simulink model "EngPrt"  (R2018a)
settings: configuration reference "cs_ert" (kept outside this file)
settings Model: DataDictionary=EngPrt.sldd  Creator=zhoutinglin  LastModifiedBy=zhoutinglin

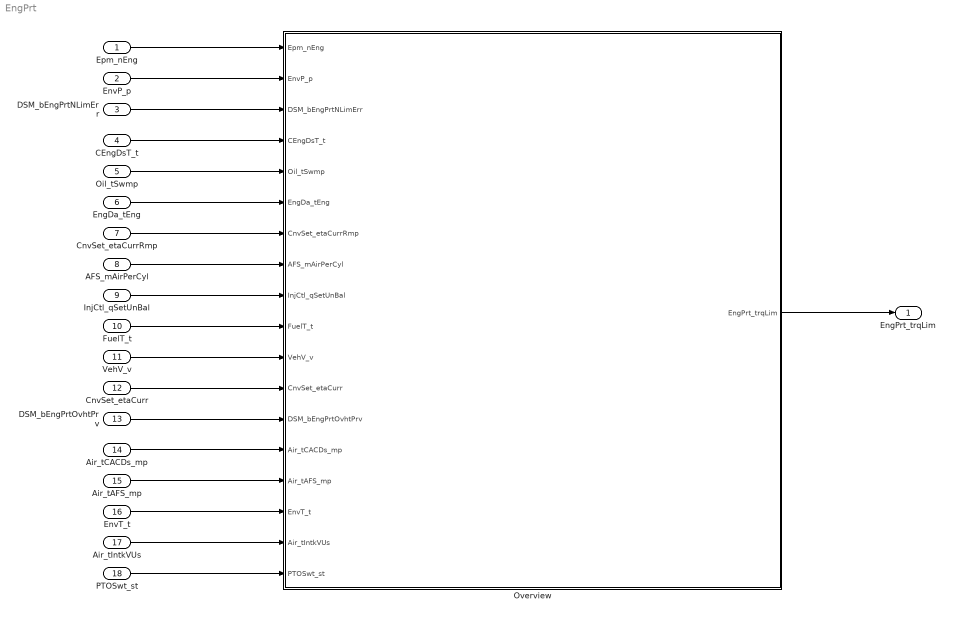
== system EngPrt ==
  Epm_nEng : Inport
  EnvP_p : Inport  Port=2
  DSM_bEngPrtNLimErr : Inport  Port=3
  CEngDsT_t : Inport  Port=4
  Oil_tSwmp : Inport  Port=5
  EngDa_tEng : Inport  Port=6
  CnvSet_etaCurrRmp : Inport  Port=7
  AFS_mAirPerCyl : Inport  Port=8
  InjCtl_qSetUnBal : Inport  Port=9
  FuelT_t : Inport  Port=10
  VehV_v : Inport  Port=11
  CnvSet_etaCurr : Inport  Port=12
  DSM_bEngPrtOvhtPrv : Inport  Port=13
  Air_tCACDs_mp : Inport  Port=14
  Air_tAFS_mp : Inport  Port=15
  EnvT_t : Inport  Port=16
  Air_tIntkVUs : Inport  Port=17
  PTOSwt_st : Inport  Port=18
  Overview : Subsystem
  EngPrt_trqLim : Outport
  wires:
  Epm_nEng/1 -> Overview/1(Epm_nEng)
  EnvP_p/1 -> Overview/2(EnvP_p)
  DSM_bEngPrtNLimErr/1 -> Overview/3(DSM_bEngPrtNLimErr)
  CEngDsT_t/1 -> Overview/4(CEngDsT_t)
  Oil_tSwmp/1 -> Overview/5(Oil_tSwmp)
  EngDa_tEng/1 -> Overview/6(EngDa_tEng)
  CnvSet_etaCurrRmp/1 -> Overview/7(CnvSet_etaCurrRmp)
  AFS_mAirPerCyl/1 -> Overview/8(AFS_mAirPerCyl)
  InjCtl_qSetUnBal/1 -> Overview/9(InjCtl_qSetUnBal)
  FuelT_t/1 -> Overview/10(FuelT_t)
  VehV_v/1 -> Overview/11(VehV_v)
  CnvSet_etaCurr/1 -> Overview/12(CnvSet_etaCurr)
  DSM_bEngPrtOvhtPrv/1 -> Overview/13(DSM_bEngPrtOvhtPrv)
  Air_tCACDs_mp/1 -> Overview/14(Air_tCACDs_mp)
  Air_tAFS_mp/1 -> Overview/15(Air_tAFS_mp)
  EnvT_t/1 -> Overview/16(EnvT_t)
  Air_tIntkVUs/1 -> Overview/17(Air_tIntkVUs)
  PTOSwt_st/1 -> Overview/18(PTOSwt_st)
  Overview/1(EngPrt_trqLim) -> EngPrt_trqLim/1

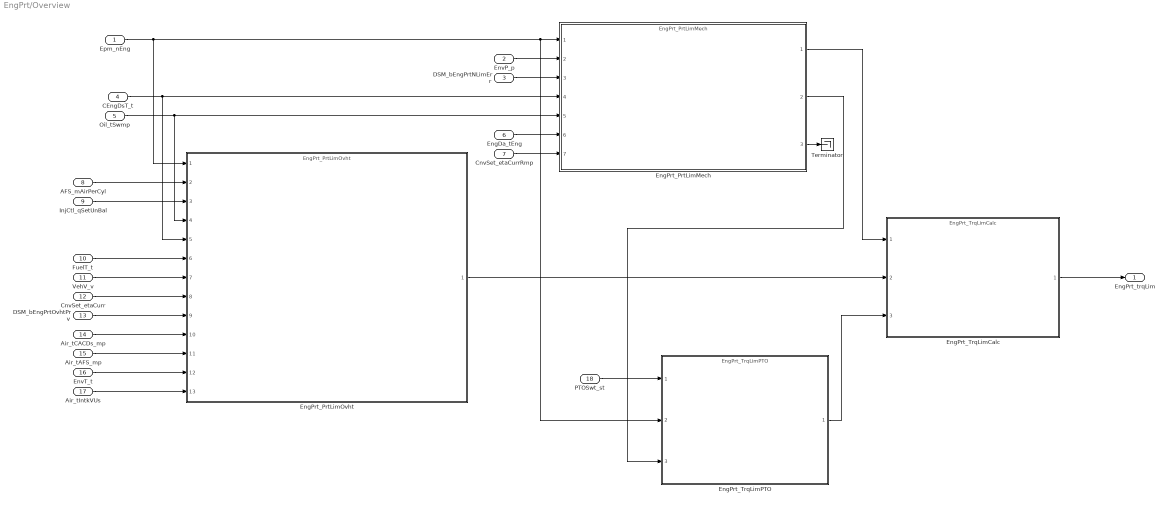
== system EngPrt/Overview ==
  Epm_nEng : Inport
  EnvP_p : Inport  Port=2
  DSM_bEngPrtNLimErr : Inport  Port=3
  CEngDsT_t : Inport  Port=4
  Oil_tSwmp : Inport  Port=5
  EngDa_tEng : Inport  Port=6
  CnvSet_etaCurrRmp : Inport  Port=7
  AFS_mAirPerCyl : Inport  Port=8
  InjCtl_qSetUnBal : Inport  Port=9
  FuelT_t : Inport  Port=10
  VehV_v : Inport  Port=11
  CnvSet_etaCurr : Inport  Port=12
  DSM_bEngPrtOvhtPrv : Inport  Port=13
  Air_tCACDs_mp : Inport  Port=14
  Air_tAFS_mp : Inport  Port=15
  EnvT_t : Inport  Port=16
  Air_tIntkVUs : Inport  Port=17
  PTOSwt_st : Inport  Port=18
  EngPrt_PrtLimMech : ModelReference  ModelNameDialog=EngPrt_PrtLimMech  SimulationMode=Normal  ModelReferenceVersion=1.55
  EngPrt_PrtLimOvht : ModelReference  ModelNameDialog=EngPrt_PrtLimOvht  SimulationMode=Normal  ModelReferenceVersion=1.64
  EngPrt_TrqLimCalc : ModelReference  ModelNameDialog=EngPrt_TrqLimCalc  SimulationMode=Normal  ModelReferenceVersion=1.49
  EngPrt_TrqLimPTO : ModelReference  ModelNameDialog=EngPrt_TrqLimPTO  SimulationMode=Normal  ModelReferenceVersion=1.49
  Terminator : Terminator
  EngPrt_trqLim : Outport
  wires:
  EngPrt_TrqLimPTO/1 -> EngPrt_TrqLimCalc/3
  EngPrt_PrtLimOvht/1 -> EngPrt_TrqLimCalc/2
  EngPrt_PrtLimMech/1 -> EngPrt_TrqLimCalc/1
  Epm_nEng/1 -> EngPrt_PrtLimOvht/1, EngPrt_TrqLimPTO/2, EngPrt_PrtLimMech/1
  EnvP_p/1 -> EngPrt_PrtLimMech/2
  DSM_bEngPrtNLimErr/1 -> EngPrt_PrtLimMech/3
  CEngDsT_t/1 -> EngPrt_PrtLimOvht/5, EngPrt_PrtLimMech/4
  Oil_tSwmp/1 -> EngPrt_PrtLimOvht/4, EngPrt_PrtLimMech/5
  EngDa_tEng/1 -> EngPrt_PrtLimMech/6
  CnvSet_etaCurrRmp/1 -> EngPrt_PrtLimMech/7
  EngPrt_PrtLimMech/2 -> EngPrt_TrqLimPTO/3
  AFS_mAirPerCyl/1 -> EngPrt_PrtLimOvht/2
  InjCtl_qSetUnBal/1 -> EngPrt_PrtLimOvht/3
  FuelT_t/1 -> EngPrt_PrtLimOvht/6
  VehV_v/1 -> EngPrt_PrtLimOvht/7
  CnvSet_etaCurr/1 -> EngPrt_PrtLimOvht/8
  DSM_bEngPrtOvhtPrv/1 -> EngPrt_PrtLimOvht/9
  Air_tCACDs_mp/1 -> EngPrt_PrtLimOvht/10
  Air_tAFS_mp/1 -> EngPrt_PrtLimOvht/11
  EnvT_t/1 -> EngPrt_PrtLimOvht/12
  Air_tIntkVUs/1 -> EngPrt_PrtLimOvht/13
  EngPrt_TrqLimCalc/1 -> EngPrt_trqLim/1
  PTOSwt_st/1 -> EngPrt_TrqLimPTO/1
  EngPrt_PrtLimMech/3 -> Terminator/1
